simulink model "simulink_double_step"  (R2024b)
settings: Solver=ode4  StartTime=0.0  StopTime=20  FixedStep=1e-3  RelTol=1e-3
undefined symbols (not defined in the file): linear_sys, sim_step_gain
settings Model: Creator=Admin  LastModifiedBy=david

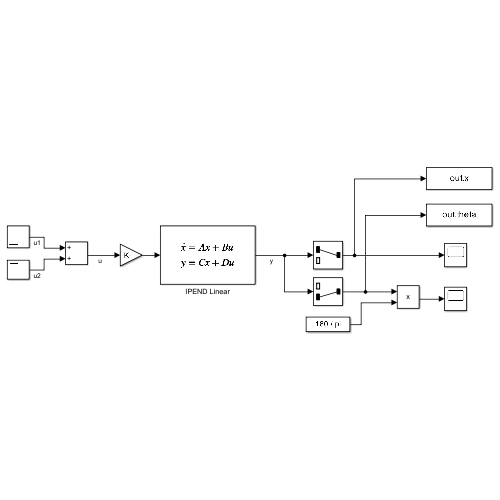
[thumbnail: Simulink's stored preview of the top-level diagram]
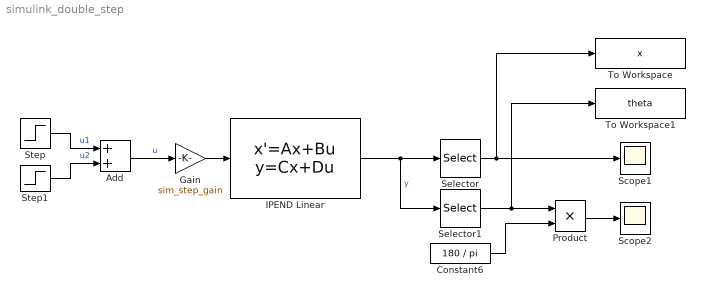
== system simulink_double_step ==
  Add : Sum
  Constant6 : Constant  Value=180 / pi
  Gain : Gain  Gain=sim_step_gain
  IPEND Linear : StateSpace  A=linear_sys.A  B=linear_sys.B  C=linear_sys.C  D=linear_sys.D  InitialCondition=[0 0 0 0]'
  Product : Product
  Scope1 : Scope
  Scope2 : Scope
  Selector : Selector  InputPortWidth=2  IndexOptions=Index vector (dialog)  Indices=1  OutputSizes=1
  Selector1 : Selector  InputPortWidth=2  IndexOptions=Index vector (dialog)  Indices=2  OutputSizes=1
  Step : Step  SampleTime=0
  Step1 : Step  Time=2  After=-1  SampleTime=0
  To Workspace : ToWorkspace  VariableName=x  SampleTime=-1
      settings: Save2DSignal=2-D array (concatenate along first dimension)
  To Workspace1 : ToWorkspace  VariableName=theta  SampleTime=-1
      settings: Save2DSignal=2-D array (concatenate along first dimension)
  wires:
  IPEND Linear/1 -> Selector/1, Selector1/1  "y"
  Step/1 -> Add/1  "u1"
  Step1/1 -> Add/2  "u2"
  Add/1 -> Gain/1  "u"
  Gain/1 -> IPEND Linear/1
  Selector1/1 -> To Workspace1/1, Product/1
  Selector/1 -> To Workspace/1, Scope1/1
  Product/1 -> Scope2/1
  Constant6/1 -> Product/2
